simulink model "vChassis"  (R2024b)
settings: configuration reference "STM32H7_Config" (kept outside this file)
undefined symbols (not defined in the file): tSystemsTask
settings Model: DataDictionary=Master_Dictionary.sldd  EnableAccessToBaseWorkspace=off  Creator=torni  LastModifiedBy=William
settings ConfigSetRef: SourceName=STM32H7_Config

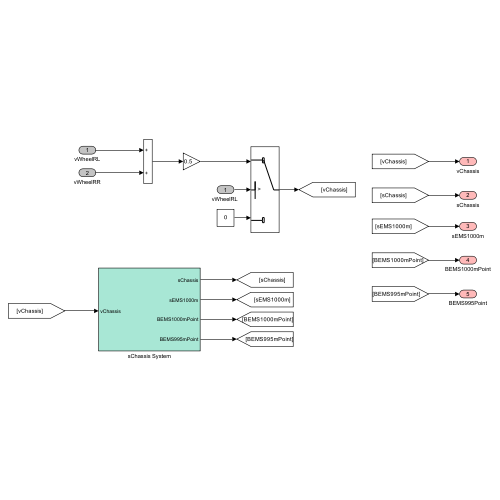
[thumbnail: Simulink's stored preview of the top-level diagram]
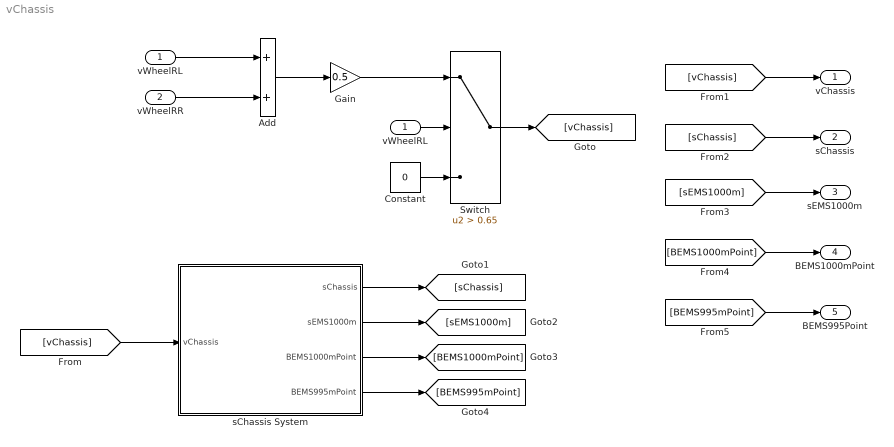
== system vChassis ==
  vWheelRL : Inport  OutDataTypeStr=double
  vWheelRR : Inport  Port=2  OutDataTypeStr=double
  Add : Sum
  Constant : Constant  Value=0
  Gain : Gain  Gain=0.5
  Switch : Switch  Criteria=u2 > Threshold  Threshold=0.65  SaturateOnIntegerOverflow=off  InputSameDT=off
  sChassis System : Subsystem
  "vWheelRL " : InportShadow  OutDataTypeStr=double
  vChassis : Outport  OutDataTypeStr=double  VectorParamsAs1DForOutWhenUnconnected=off
  sChassis : Outport  Port=2  OutDataTypeStr=double  VectorParamsAs1DForOutWhenUnconnected=off
  sEMS1000m : Outport  Port=3  OutDataTypeStr=double  VectorParamsAs1DForOutWhenUnconnected=off
  BEMS1000mPoint : Outport  Port=4  OutDataTypeStr=boolean  VectorParamsAs1DForOutWhenUnconnected=off
  BEMS995Point : Outport  Port=5  OutDataTypeStr=boolean  VectorParamsAs1DForOutWhenUnconnected=off
  wires:
  vWheelRL/1 -> Add/1
  vWheelRR/1 -> Add/2
  [vChassis] -> sChassis System/1(vChassis)
  sChassis System/1(sChassis) -> [sChassis]
  [vChassis] -> vChassis/1
  [sChassis] -> sChassis/1
  Gain/1 -> Switch/1
  "vWheelRL "/1 -> Switch/2
  Constant/1 -> Switch/3
  Switch/1 -> [vChassis]
  sChassis System/2(sEMS1000m) -> [sEMS1000m]
  sChassis System/3(BEMS1000mPoint) -> [BEMS1000mPoint]
  sChassis System/4(BEMS995mPoint) -> [BEMS995mPoint]
  [BEMS1000mPoint] -> BEMS1000mPoint/1
  [sEMS1000m] -> sEMS1000m/1
  [BEMS995mPoint] -> BEMS995Point/1
  Add/1 -> Gain/1

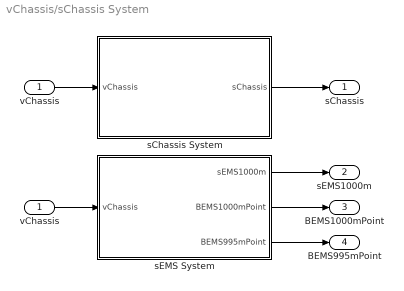
== system vChassis/sChassis System ==
  vChassis : Inport  OutDataTypeStr=double
  sChassis System : Subsystem
  sEMS System : Subsystem
  "vChassis  " : InportShadow  OutDataTypeStr=double
  sChassis : Outport  OutDataTypeStr=double  VectorParamsAs1DForOutWhenUnconnected=off
  sEMS1000m : Outport  Port=2  OutDataTypeStr=double  VectorParamsAs1DForOutWhenUnconnected=off
  BEMS1000mPoint : Outport  Port=3  OutDataTypeStr=boolean  VectorParamsAs1DForOutWhenUnconnected=off
  BEMS995mPoint : Outport  Port=4  OutDataTypeStr=boolean  VectorParamsAs1DForOutWhenUnconnected=off
  wires:
  sEMS System/1(sEMS1000m) -> sEMS1000m/1
  sEMS System/2(BEMS1000mPoint) -> BEMS1000mPoint/1
  sEMS System/3(BEMS995mPoint) -> BEMS995mPoint/1
  "vChassis  "/1 -> sEMS System/1(vChassis)
  vChassis/1 -> sChassis System/1(vChassis)
  sChassis System/1(sChassis) -> sChassis/1

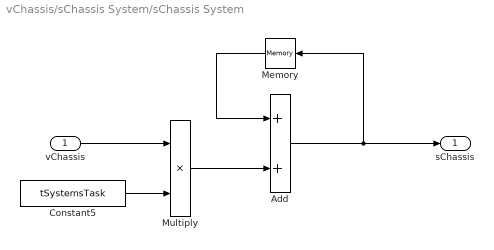
== system vChassis/sChassis System/sChassis System ==
  vChassis : Inport  OutDataTypeStr=double
  Add : Sum
  Constant5 : Constant  Value=tSystemsTask
  Memory : Memory  InheritSampleTime=on
  Multiply : Product
  sChassis : Outport  OutDataTypeStr=double  VectorParamsAs1DForOutWhenUnconnected=off
  wires:
  Constant5/1 -> Multiply/2
  Add/1 -> sChassis/1, Memory/1
  vChassis/1 -> Multiply/1
  Memory/1 -> Add/1
  Multiply/1 -> Add/2

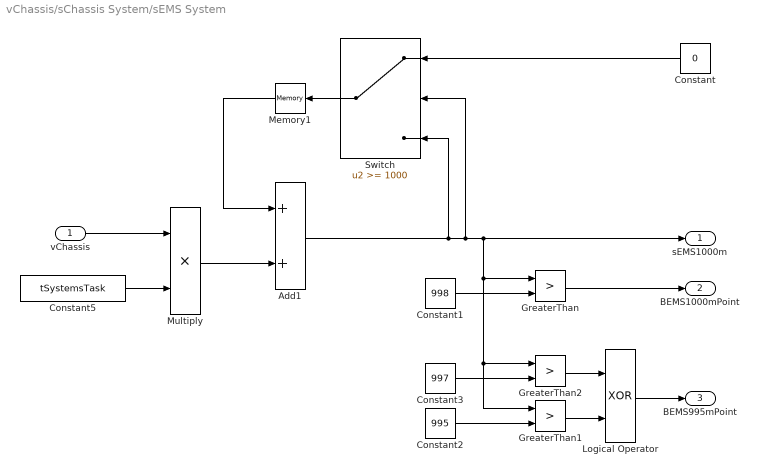
== system vChassis/sChassis System/sEMS System ==
  vChassis : Inport  OutDataTypeStr=double
  Add1 : Sum
  Constant : Constant  Value=0
  Constant1 : Constant  Value=998
  Constant2 : Constant  Value=995
  Constant3 : Constant  Value=997
  Constant5 : Constant  Value=tSystemsTask
  GreaterThan : RelationalOperator  Operator=>  OutDataTypeStr=boolean  RndMeth=Simplest  InputSameDT=off
  GreaterThan1 : RelationalOperator  Operator=>  OutDataTypeStr=boolean  RndMeth=Simplest  InputSameDT=off
  GreaterThan2 : RelationalOperator  Operator=>  OutDataTypeStr=boolean  RndMeth=Simplest  InputSameDT=off
  Logical Operator : Logic  Operator=XOR  AllPortsSameDT=off  OutDataTypeStr=boolean
  Memory1 : Memory  InheritSampleTime=on
  Multiply : Product
  Switch : Switch  Threshold=1000  SaturateOnIntegerOverflow=off  InputSameDT=off
  sEMS1000m : Outport  OutDataTypeStr=double  VectorParamsAs1DForOutWhenUnconnected=off
  BEMS1000mPoint : Outport  Port=2  OutDataTypeStr=boolean  VectorParamsAs1DForOutWhenUnconnected=off
  BEMS995mPoint : Outport  Port=3  OutDataTypeStr=boolean  VectorParamsAs1DForOutWhenUnconnected=off
  wires:
  GreaterThan/1 -> BEMS1000mPoint/1
  Add1/1 -> GreaterThan2/1, GreaterThan1/1, GreaterThan/1, sEMS1000m/1, Switch/2, Switch/3
  GreaterThan1/1 -> Logical Operator/2
  Constant1/1 -> GreaterThan/2
  Constant2/1 -> GreaterThan1/2
  Memory1/1 -> Add1/1
  Logical Operator/1 -> BEMS995mPoint/1
  Constant3/1 -> GreaterThan2/2
  Constant/1 -> Switch/1
  Switch/1 -> Memory1/1
  GreaterThan2/1 -> Logical Operator/1
  Multiply/1 -> Add1/2
  vChassis/1 -> Multiply/1
  Constant5/1 -> Multiply/2
